simulink model "pilot2d"  (R2022b)
settings: Solver=VariableStepAuto  StartTime=0.0  StopTime=10  RelTol=1e-3
libraries: sim3dlib x1, uavsim3dlib x1, aerolibanimutils x1, simulink x1
settings Model: Creator=l.ribeiro-lustosa  LastModifiedBy=fades
settings DebuggingCC: UnconnectedInputMsg=warning  UnconnectedOutputMsg=warning  UnconnectedLineMsg=warning
settings ModelReferenceCC: EnableRefExpFcnMdlSchedulingChecks=on
settings RTWCC: DLArmComputeVersion=19.05

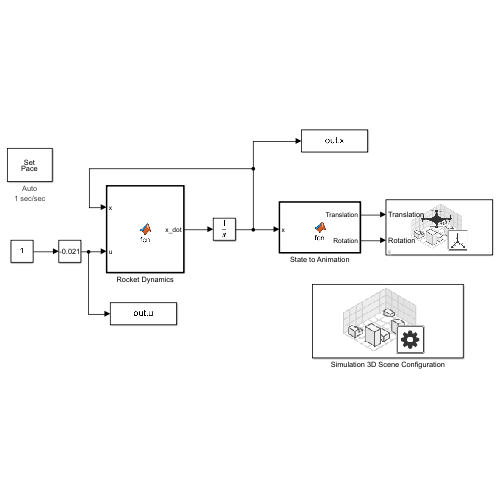
[thumbnail: Simulink's stored preview of the top-level diagram]
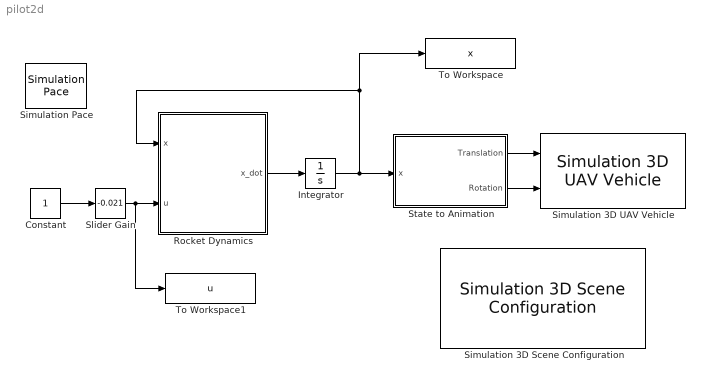
== system pilot2d ==
  Constant : Constant  SampleTime=0.02
  Integrator : Integrator  InitialCondition=[0 -1 0 0 0 0]
  Rocket Dynamics : MATLAB Function  TreatAsAtomicUnit=on
  Simulation 3D Scene Configuration : sim3dlib/Simulation 3D Scene Configuration  Priority=0  ProjectFormat=Default Scenes  SceneDesc=US city block  ProjectName=D:\MATLAB\toolbox\shared\sim3d_projects\automotive_project\UE4\WindowsNoEditor\VehicleSimulation.exe  ScenePath=/Game/Maps/USCityBlock  EnableOpenDRIVE=off  vehTagList={'Rocket';'Scene Origin'}  vehTag=Rocket  OpVisEn=off  Ts=0.02  EnableWindow=on  EnableRemoteAccess=off  EnableWeather=off  SunAltitude=40.0  SunAzimuth=90  clouds=10  wind=1  fog=0  rain=0  EnableGeospatial=off  OriginHeight=200  OriginLatitude=40.744652  OriginLongitude=-73.988864  MapStyle=Aerial  AdditionalAssetIDs=[]  UseAdvancedSunSky=off  SolarTime=11  TimeZone=-5  Day=21  Month=9  Year=2022  UseDaylightSavingTime=on  DSTStartDay=10  DSTStartMonth=3  DSTEndDay=3  DSTEndMonth=11  DSTSwitchHour=2  sensorTag=MainCamera1  sensorId=1  sensorName=MainCamera1  mountLoc=Origin  offsetFlag=off  tmountOffset=[0, 0, 0]  rmountOffset=[0, 0, 0]  HorizontalResolution=1280  VerticalResolution=720  HorizontalFOV=60  mountPoint=[0 0 0]  mountOrientation=[0 0 0]  aMode=4  ID=1  GeoTrigger=Inactive
  Simulation 3D UAV Vehicle : uavsim3dlib/Simulation 3D UAV Vehicle  Priority=-1  Mesh=Quadrotor  MeshPath=/MathWorksUAVContent/UAVs/HexaRotorUAV/HexaRotor.HexaRotor  Color=Black  ActorName=Rocket  InitialTranslation=[0 0 1]  InitialRotation=[0 0 0]  SampleTime=-1  ActorType=SimulinkVehicle  ID=C  aMode=4  ActorTag=Rocket
  Simulation Pace : aerolibanimutils/Simulation Pace  SimulationPace=1  SleepMode=Auto  OutputPaceError=off  SampleTime=0.02
  Slider Gain : simulink/Math Operations/Slider Gain  gain=-0.021  low=-0.1745  high=0.1745
  State to Animation : MATLAB Function  TreatAsAtomicUnit=on
  To Workspace : ToWorkspace  VariableName=x  SaveFormat=Timeseries  SampleTime=-1
  To Workspace1 : ToWorkspace  VariableName=u  SaveFormat=Timeseries  SampleTime=-1
  wires:
  Rocket Dynamics/1(x_dot) -> Integrator/1
  Integrator/1 -> State to Animation/1(x), To Workspace/1, Rocket Dynamics/1(x)
  State to Animation/1(Translation) -> Simulation 3D UAV Vehicle/1
  State to Animation/2(Rotation) -> Simulation 3D UAV Vehicle/2
  Slider Gain/1 -> To Workspace1/1, Rocket Dynamics/2(u)
  Constant/1 -> Slider Gain/1

== matlab function pilot2d/State to Animation ==
  data: x input; Translation output; Rotation output
function [Translation,Rotation] = fcn(x)

Translation = [ x(1) 0 -x(2) ]';
Rotation = [ 0 x(5) 0 ]';

== matlab function pilot2d/Rocket Dynamics ==
  data: x input; x_dot output; u input
function x_dot = fcn(x,u)

%% rocket params
m = 0.2;
h_cg = 0.5;
J = 1/12*m*(h_cg*2)^2; % using 1/12ML^2 formula
g = 10;
T = m*g*1.0;

%% init variables
x_dot = zeros(6,1);
the = x(5);
del = u(1);

%% derivative of position is velocity
x_dot(1:2) = x(3:4);

%% derivative of velocity
x_dot(3:4) = -[ sin(del+the); cos(del+the)]*T/m + [0;1]*g;

%% derivative of angle
x_dot(5) = x(6);

%% derivative of angular velocity
M = -T*h_cg*sin(del);
x_dot(6) = 1/J*M;
